simulink model "mfbase"  (R2025a)
settings: Solver=VariableStepAuto  StartTime=0.0  StopTime=7.5  RelTol=1e-3
values from neighbouring files (symbols this model uses):
  Accen = 0    [desm1210_boif1302_analogique.m]
  Bruit = 0    [desm1210_boif1302_analogique.m]
undefined symbols (not defined in the file or in its folder): dspblkCoreblockFVToolHelper, gcbh
libraries: dspfdesign x5, dspobslib x2, dspsigops x2, commanapbnd3 x1, dspsrcs4 x1
settings Model: Creator=sebastienroy  LastModifiedBy=francoisdesautels
settings SolverCC: AlgebraicLoopSolver=TrustRegion
settings DebuggingCC: UnconnectedInputMsg=warning  UnconnectedOutputMsg=warning  UnconnectedLineMsg=warning
settings ModelReferenceCC: EnableRefExpFcnMdlSchedulingChecks=on
settings RTWCC: GPUComputeCapability=3.5  DLArmComputeVersion=19.05

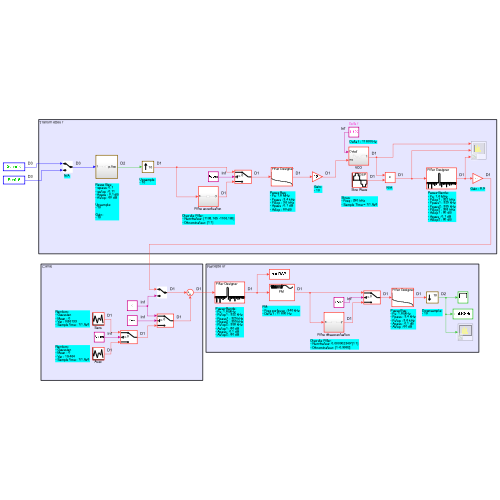
[thumbnail: Simulink's stored preview of the top-level diagram]
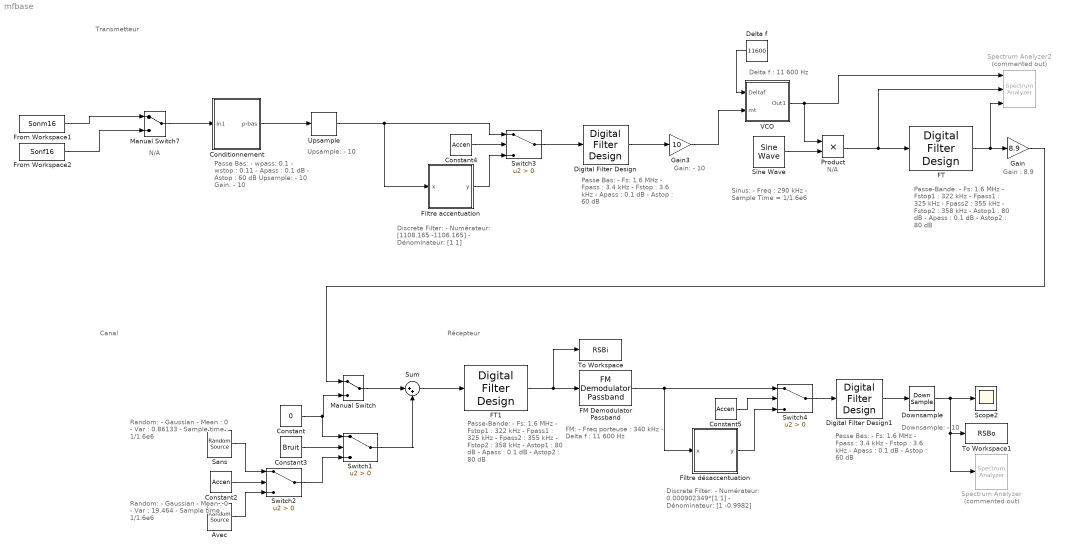
== system mfbase ==
  note: Discrete Filter:
      | - Numérateur: [1108.165 -1106.165]
      | - Dénominateur: [1 1]
  note: Passe Bas:
      | - wpass: 0.1
      | - wstop : 0.11
      | - Apass : 0.1 dB
      | - Astop : 60 dB
      |
      | Upsample:
      | - 10
      |
      | Gain:
      | - 10
  note: Transmetteur
  note: Récepteur
  note: Canal
  note: N/A
  note: N/A
  note: Upsample:
      | - 10
  note: Passe Bas:
      | - Fs: 1.6 MHz
      | - Fpass : 3.4 kHz
      | - Fstop : 3.6 kHz
      | - Apass : 0.1 dB
      | - Astop : 60 dB
  note: Gain:
      | - 10
  note: Sinus:
      | - Freq : 290 kHz
      | - Sample Time = 1/1.6e6
  note: Passe-Bande:
      | - Fs: 1.6 MHz
      | - Fstop1 : 322 kHz
      | - Fpass1 : 325 kHz
      | - Fpass2 : 355 kHz
      | - Fstop2 : 358 kHz
      | - Astop1 : 80 dB
      | - Apass : 0.1 dB
      | - Astop2 : 80 dB
  note: Passe-Bande:
      | - Fs: 1.6 MHz
      | - Fstop1 : 322 kHz
      | - Fpass1 : 325 kHz
      | - Fpass2 : 355 kHz
      | - Fstop2 : 358 kHz
      | - Astop1 : 80 dB
      | - Apass : 0.1 dB
      | - Astop2 : 80 dB
  note: Random:
      | - Gaussian
      | - Mean : 0
      | - Var : 0.86133
      | - Sample time : 1/1.6e6
  note: Random:
      | - Gaussian
      | - Mean : 0
      | - Var : 19.464
      | - Sample time : 1/1.6e6
  note: FM:
      | - Freq porteuse : 340 kHz
      | - Delta f : 11 600 Hz
  note: Passe Bas:
      | - Fs: 1.6 MHz
      | - Fpass : 3.4 kHz
      | - Fstop : 3.6 kHz
      | - Apass : 0.1 dB
      | - Astop : 60 dB
  note: Discrete Filter:
      | - Numérateur: 0.000902349*[1 1]
      | - Dénominateur: [1 -0.9982]
  note: Downsample:
      | - 10
  note: Delta f : 11 600 Hz
  note: Gain : 8.9
  Avec : dspobslib/Random Source  SrcType=Gaussian  NormMethod=Ziggurat  CltLength=12  MinVal=0  MaxVal=1  MeanVal=0  VarVal=(12.165e-6)*(1.6e6)  RepMode=Not repeatable  rawSeed=1  IsInherit=off  SampMode=Discrete  SampTime=1/(1.6e6)  SampFrame=1  DataType=Double  OutComplex=Real  OutputFrames=off
  Conditionnement : Subsystem
  Constant : Constant  Value=0
  Constant2 : Constant  Value=Accen
  Constant3 : Constant  Value=Bruit
  Constant4 : Constant  Value=Accen
  Constant5 : Constant  Value=Accen
  Delta f : Constant  Value=11600
  Digital Filter Design : dspfdesign/Digital Filter Design  mwdsp_browser_bugfix_var=off
  Digital Filter Design1 : dspfdesign/Digital Filter Design  mwdsp_browser_bugfix_var=off
  Downsample : DownSample  N=10  RateOptions=Allow multirate processing
  FM Demodulator Passband : commanapbnd3/FM Demodulator Passband  Fc=340000  Ph=0  Kc=11600  Ho=100
  FT : dspfdesign/Digital Filter Design  mwdsp_browser_bugfix_var=off
  FT1 : dspfdesign/Digital Filter Design  mwdsp_browser_bugfix_var=off
  Filtre accentuation : Subsystem
  Filtre désaccentuation : Subsystem
  From Workspace1 : FromWorkspace  VariableName=Sonm16  SampleTime=1/16000  Interpolate=off  OutputAfterFinalValue=Setting to zero
  From Workspace2 : FromWorkspace  VariableName=Sonf16  SampleTime=1/16000  Interpolate=off  OutputAfterFinalValue=Setting to zero
  Gain : Gain  Gain=8.9
  Gain3 : Gain  Gain=10
  Manual Switch : ManualSwitch
  Manual Switch7 : ManualSwitch
  Product : Product
  Sans : dspobslib/Random Source  SrcType=Gaussian  NormMethod=Ziggurat  CltLength=12  MinVal=0  MaxVal=1  MeanVal=0  VarVal=(538.33e-9)*(1.6e6)  RepMode=Not repeatable  rawSeed=1  IsInherit=off  SampMode=Discrete  SampTime=1/(1.6e6)  SampFrame=1  DataType=Double  OutComplex=Real  OutputFrames=off
  Scope2 : Scope
      settings: ActiveDisplayYMinimum=-41.036446146941891  ActiveDisplayYMaximum=5.3144262558337489  DataLoggingVariableName=ScopeData2
  Sine Wave : dspsrcs4/Sine Wave  Amplitude=1  Frequency=290000  Phase=0  SampleMode=Discrete  OutComplex=Real  CompMethod=Trigonometric fcn  TableSize=Speed  SampleTime=1/(1.6e6)  SamplesPerFrame=1  ResetState=Restart at time zero  OutputFrames=off  dataType=double  wordLen=16  udDataType=sfix(16)  fracBitsMode=Best precision  numFracBits=15  OutDataTypeStr=double  LastOutDataTypeStr=double
  Spectrum Analyzer : SpectrumAnalyzer  Commented=on  WindowPosition=[1.000000,1.000000,2056.000000,1257.000000,]  ScopeFrameLocation=window  SpectrumType=Power density  WindowInvariantSamplesPerUpdate=on  SpectrumUnits=dBm/Hz  YLimits=[-147.624 -5.1467]
  Spectrum Analyzer2 : SpectrumAnalyzer  Commented=on  NumInputPorts=3  WindowPosition=[1.000000,1.000000,2056.000000,1257.000000,]  ScopeFrameLocation=window  SpectrumType=Power density  Method=Welch  SampleRate=1600000  AxesScaling=Manual  FFTLength=128  Span=1000000  StartFrequency=-500000  StopFrequency=500000  OverlapPercent=80  AveragingMethod=Running  SpectralAverages=10  SpectrumUnits=dBm/Hz  YLimits=[-221.85 11.4946]  ShowLegend=on  SelectedToolstripTab=spectrumAnalyzerToolstrip.measurementsTab  MeasurementChannel=2  AllowFFTLengthLessThanSamplesPerUpdate=on  DefaultConfigurationName=spbscopes.SpectrumAnalyzerBlockCfg  IsFrequencyInputMode=0  FrequencyVectorPort=0  FrequencyVectorFromPort=0  FrequencyInputRBWPort=0  FrequencyInputRBWFromPort=0
  Sum : Sum  Inputs=|++
  Switch{1..4} (4 alike) : Switch  Criteria=u2 > Threshold  SaturateOnIntegerOverflow=off  InputSameDT=off
  To Workspace : ToWorkspace  VariableName=RSBi  SampleTime=-1
      settings: Save2DSignal=2-D array (concatenate along first dimension)
  To Workspace1 : ToWorkspace  VariableName=RSBo  SampleTime=-1
      settings: Save2DSignal=2-D array (concatenate along first dimension)
  Upsample : dspsigops/Upsample  FactorSource=Dialog parameter  N=10  Nmax=16  phase=0  RateOptions=Allow multirate processing  ic=0  mode=Unused parameter value
  VCO : Subsystem
  wires:
  FT/1 -> Spectrum Analyzer2/3, Gain/1
  Product/1 -> Spectrum Analyzer2/2, FT/1
  Sine Wave/1 -> Product/2
  VCO/1(Out1) -> Spectrum Analyzer2/1, Product/1
  Digital Filter Design/1 -> Gain3/1
  Switch2/1 -> Switch1/3
  Constant4/1 -> Switch3/2
  Constant5/1 -> Switch4/2
  Filtre accentuation/1(y) -> Switch3/3
  Conditionnement/1(p-bas) -> Upsample/1
  Switch3/1 -> Digital Filter Design/1
  Downsample/1 -> To Workspace1/1, Spectrum Analyzer/1, Scope2/1
  Manual Switch/1 -> Sum/1
  Constant3/1 -> Switch1/2
  Switch4/1 -> Digital Filter Design1/1
  Manual Switch7/1 -> Conditionnement/1(In1)
  Constant/1 -> Switch1/1, Manual Switch/2
  FM Demodulator Passband/1 -> Filtre désaccentuation/1(x), Switch4/1
  Gain/1 -> Manual Switch/1
  Gain3/1 -> VCO/2(mt)
  Avec/1 -> Switch2/3
  Sans/1 -> Switch2/1
  Switch1/1 -> Sum/2
  Constant2/1 -> Switch2/2
  Digital Filter Design1/1 -> Downsample/1
  FT1/1 -> To Workspace/1, FM Demodulator Passband/1
  Delta f/1 -> VCO/1("Deltaf ")
  Upsample/1 -> Filtre accentuation/1(x), Switch3/1
  Filtre désaccentuation/1(y) -> Switch4/3
  From Workspace1/1 -> Manual Switch7/1
  From Workspace2/1 -> Manual Switch7/2
  Sum/1 -> FT1/1

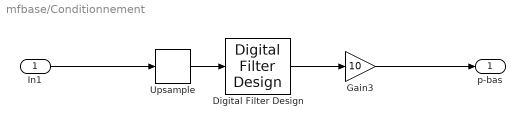
== system mfbase/Conditionnement ==
  In1 : Inport
  Digital Filter Design : dspfdesign/Digital Filter Design  mwdsp_browser_bugfix_var=off
  Gain3 : Gain  Gain=10
  Upsample : dspsigops/Upsample  FactorSource=Dialog parameter  N=10  Nmax=16  phase=0  RateOptions=Allow multirate processing  ic=0  mode=Unused parameter value
  p-bas : Outport
  wires:
  Upsample/1 -> Digital Filter Design/1
  Digital Filter Design/1 -> Gain3/1
  In1/1 -> Upsample/1
  Gain3/1 -> p-bas/1

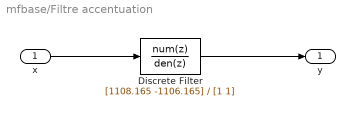
== system mfbase/Filtre accentuation ==
  x : Inport
  Discrete Filter : DiscreteFilter  LoadFcn=dspblkCoreblockFVToolHelper(gcbh,'load');  Numerator=[1108.165 -1106.165]  Denominator=[1 1]
      settings: CopyFcn=dspblkCoreblockFVToolHelper(gcbh,'copy');  DeleteFcn=dspblkCoreblockFVToolHelper(gcbh,'close');  ModelCloseFcn=dspblkCoreblockFVToolHelper(gcbh,'close');  PreSaveFcn=dspblkCoreblockFVToolHelper(gcbh,'presave');  PostSaveFcn=dspblkCoreblockFVToolHelper(gcbh,'postsave');  CloseFcn=dspblkCoreblockFVToolHelper(gcbh,'close');
  y : Outport
  wires:
  x/1 -> Discrete Filter/1
  Discrete Filter/1 -> y/1

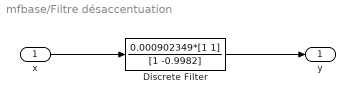
== system mfbase/Filtre désaccentuation ==
  x : Inport
  Discrete Filter : DiscreteFilter  LoadFcn=dspblkCoreblockFVToolHelper(gcbh,'load');  Numerator=0.000902349*[1 1]  Denominator=[1 -0.9982]
      settings: CopyFcn=dspblkCoreblockFVToolHelper(gcbh,'copy');  DeleteFcn=dspblkCoreblockFVToolHelper(gcbh,'close');  ModelCloseFcn=dspblkCoreblockFVToolHelper(gcbh,'close');  PreSaveFcn=dspblkCoreblockFVToolHelper(gcbh,'presave');  PostSaveFcn=dspblkCoreblockFVToolHelper(gcbh,'postsave');  CloseFcn=dspblkCoreblockFVToolHelper(gcbh,'close');
  y : Outport
  wires:
  x/1 -> Discrete Filter/1
  Discrete Filter/1 -> y/1

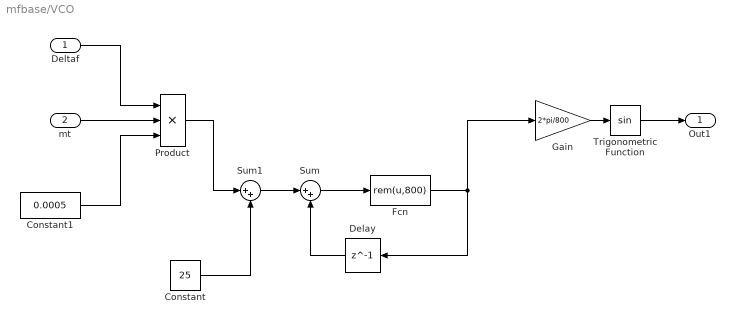
== system mfbase/VCO ==
  "Deltaf " : Inport
  mt : Inport  Port=2
  Constant : Constant  Value=25
  Constant1 : Constant  Value=0.0005
  Delay : Delay  DelayLength=1  InitialCondition=0
  Fcn : Fcn  Expr=rem(u,800)
  Gain : Gain  Gain=2*pi/800
  Product : Product  Inputs=3
  Sum : Sum  Inputs=|++
  Sum1 : Sum  Inputs=|++
  Trigonometric Function : Trigonometry
  Out1 : Outport
  wires:
  Delay/1 -> Sum/2
  Sum/1 -> Fcn/1
  Fcn/1 -> Gain/1, Delay/1
  Gain/1 -> Trigonometric Function/1
  Trigonometric Function/1 -> Out1/1
  "Deltaf "/1 -> Product/1
  mt/1 -> Product/2
  Constant1/1 -> Product/3
  Sum1/1 -> Sum/1
  Constant/1 -> Sum1/2
  Product/1 -> Sum1/1
